simulink model "Problem4"  (R2020b)
settings: Solver=VariableStepAuto  StartTime=0.0  StopTime=10.0  RelTol=1e-3
values from neighbouring files (symbols this model uses):
  b = 3.5077e-6    (= 3.5077e-06)    [Parameters.m]
  J = 3.2284e-6    (= 3.2284e-06)    [Parameters.m]
  L = 2.75e-6    (= 2.75e-06)    [Parameters.m]
  R = 4    [Parameters.m]
undefined symbols (not defined in the file or in its folder): K0, K1
settings Model: Creator=Dell  LastModifiedBy=Dell

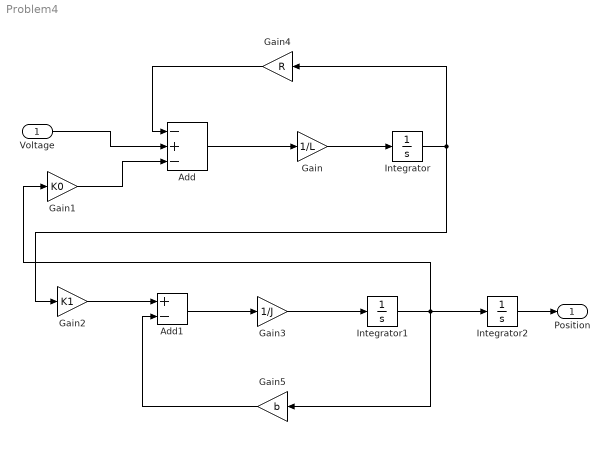
== system Problem4 ==
  Voltage : Inport
  Add : Sum  Inputs=-+-
  Add1 : Sum  Inputs=+-
  Gain : Gain  Gain=1/L
  Gain1 : Gain  Gain=K0
  Gain2 : Gain  Gain=K1
  Gain3 : Gain  Gain=1/J
  Gain4 : Gain  Gain=R
  Gain5 : Gain  Gain=b
  Integrator : Integrator
  Integrator1 : Integrator
  Integrator2 : Integrator
  Position : Outport
  wires:
  Integrator2/1 -> Position/1
  Gain2/1 -> Add1/1
  Gain3/1 -> Integrator1/1
  Add1/1 -> Gain3/1
  Gain5/1 -> Add1/2
  Integrator1/1 -> Gain5/1, Gain1/1, Integrator2/1
  Gain1/1 -> Add/3
  Voltage/1 -> Add/2
  Gain4/1 -> Add/1
  Integrator/1 -> Gain2/1, Gain4/1
  Gain/1 -> Integrator/1
  Add/1 -> Gain/1
